simulink model "AGC"  (R2021a)
settings: Solver=FixedStepAuto  StartTime=0.0  StopTime=400  RelTol=1e-3  EnableMultiTasking=on
model workspace (MAT data in the model file):
  th = 0
libraries: dspsrcs4 x2, hdlsllib x1
settings Model: EnablePacing=on  Creator=guido  LastModifiedBy=guido
settings DataIOCC: ExternalInput=x_ts
settings OptimizationCC: BlockReduction=off  ConditionallyExecuteInputs=off  DefaultParameterBehavior=Inlined
settings DebuggingCC: SignalRangeChecking=warning  AlgebraicLoopMsg=error  SingleTaskRateTransMsg=error
settings HardwareCC: ProdBitPerPointer=32  ProdBitPerSizeT=32  ProdBitPerPtrDiffT=32  ProdLargestAtomicFloat=None  ProdIntDivRoundTo=Undefined  ProdEndianess=Unspecified  ProdWordSize=32  ProdHWDeviceType=ASIC/FPGA->ASIC/FPGA  TargetBitPerPointer=64  TargetBitPerSizeT=64  TargetBitPerPtrDiffT=64  TargetLongLongMode=on  TargetIntDivRoundTo=Zero  TargetEndianess=LittleEndian  TargetWordSize=64  TargetHWDeviceType=Custom Processor->MATLAB Host Computer  ProdEqTarget=off

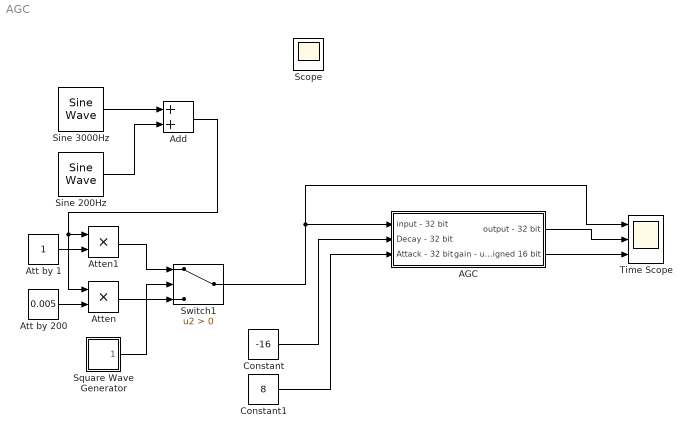
== system AGC ==
  AGC : Subsystem
  Add : Sum  AccumDataTypeStr=int32  OutDataTypeStr=int32
  Att by 1 : Constant
  Att by 200 : Constant  Value=0.005
  Atten : Product  OutDataTypeStr=int32
  Atten1 : Product  OutDataTypeStr=int32
  Constant : Constant  Value=-16  OutDataTypeStr=int32
  Constant1 : Constant  Value=8  OutDataTypeStr=int32
  Sine 200Hz : dspsrcs4/Sine Wave  Amplitude=1073741824  Frequency=200  Phase=0  SampleMode=Discrete  OutComplex=Real  CompMethod=Table lookup  TableSize=Speed  SampleTime=1/48000  SamplesPerFrame=1  ResetState=Restart at time zero  OutputFrames=off  dataType=Fixed-point  wordLen=31  udDataType=sfix(16)  fracBitsMode=Best precision  numFracBits=15  OutDataTypeStr=fixdt(1,31)  LastOutDataTypeStr=fixdt(1,31)
  Sine 3000Hz : dspsrcs4/Sine Wave  Amplitude=1073741824  Frequency=3000  Phase=0  SampleMode=Discrete  OutComplex=Real  CompMethod=Table lookup  TableSize=Speed  SampleTime=1/48000  SamplesPerFrame=1  ResetState=Restart at time zero  OutputFrames=off  dataType=Fixed-point  wordLen=31  udDataType=sfix(16)  fracBitsMode=Best precision  numFracBits=15  OutDataTypeStr=fixdt(1,31)  LastOutDataTypeStr=fixdt(1,31)
  Square Wave Generator : Subsystem  Tag=DecoupledSystem
  Switch1 : Switch  Criteria=u2 > Threshold  OutDataTypeStr=int32
  Time Scope : Scope  NumInputPorts=3
  Scope : Scope
  wires:
  Switch1/1 -> Time Scope/1, AGC/1(input - 32 bit)
  Sine 3000Hz/1 -> Add/1
  Sine 200Hz/1 -> Add/2
  Atten/1 -> Switch1/3
  Att by 200/1 -> Atten/2
  Square Wave Generator/1(Out1) -> Switch1/2
  Add/1 -> Atten1/1, Atten/1
  AGC/1(output - 32 bit) -> Time Scope/2
  AGC/2(gain - unsigned 16 bit) -> Time Scope/3
  Constant/1 -> AGC/2(Decay - 32 bit)
  Constant1/1 -> AGC/3(Attack - 32 bit)
  Atten1/1 -> Switch1/1
  Att by 1/1 -> Atten1/2

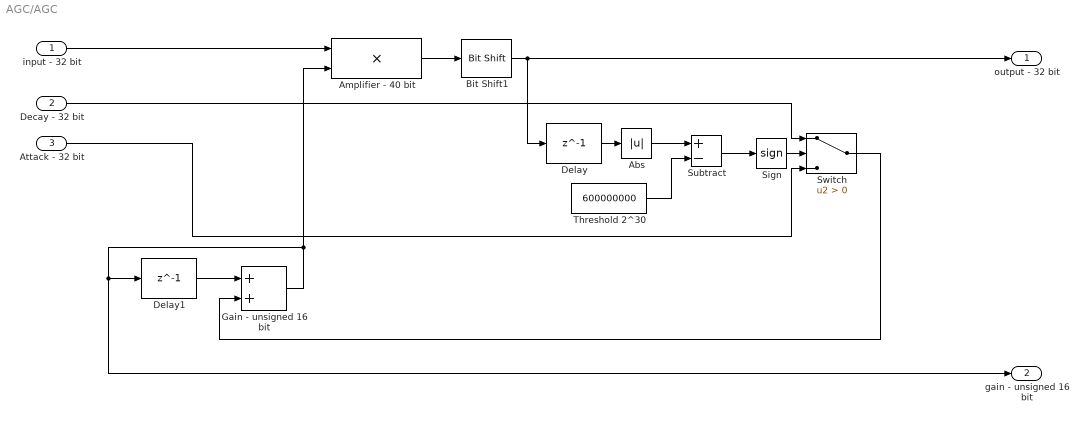
== system AGC/AGC ==
  input - 32 bit : Inport
  Decay - 32 bit : Inport  Port=2
  Attack - 32 bit : Inport  Port=3
  Abs : Abs  OutDataTypeStr=int32  SaturateOnIntegerOverflow=on
  Amplifier - 40 bit : Product  OutDataTypeStr=fixdt(1,40,0)  SaturateOnIntegerOverflow=on
  Bit Shift1 : hdlsllib/Logic and Bit Operations/Bit Shift  mode=Shift Right Arithmetic  N=8
  Delay : Delay  DelayLength=1  InitialCondition=0  UseCircularBuffer=on
  Delay1 : Delay  DelayLength=1  InitialCondition=1  UseCircularBuffer=on
  Gain - unsigned 16 bit : Sum  OutDataTypeStr=fixdt(0,16,0)  SaturateOnIntegerOverflow=on
  Sign : Signum
  Subtract : Sum  Inputs=+-  AccumDataTypeStr=int32  OutDataTypeStr=int32  SaturateOnIntegerOverflow=on
  Switch : Switch  Criteria=u2 > Threshold  OutDataTypeStr=int32  SaturateOnIntegerOverflow=on
  Threshold 2^30 : Constant  Value=600000000  OutDataTypeStr=int32
  output - 32 bit : Outport
  gain - unsigned 16 bit : Outport  Port=2
  wires:
  Delay/1 -> Abs/1
  Gain - unsigned 16 bit/1 -> Amplifier - 40 bit/2, Delay1/1, gain - unsigned 16 bit/1
  Switch/1 -> Gain - unsigned 16 bit/2
  Abs/1 -> Subtract/1
  Sign/1 -> Switch/2
  Attack - 32 bit/1 -> Switch/3
  Subtract/1 -> Sign/1
  Amplifier - 40 bit/1 -> Bit Shift1/1
  Decay - 32 bit/1 -> Switch/1
  Threshold 2^30/1 -> Subtract/2
  Delay1/1 -> Gain - unsigned 16 bit/1
  Bit Shift1/1 -> Delay/1, output - 32 bit/1
  input - 32 bit/1 -> Amplifier - 40 bit/1

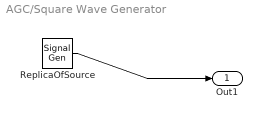
== system AGC/Square Wave Generator ==
  ReplicaOfSource : SignalGenerator  WaveForm=square  Amplitude=256  Frequency=0.5
  Out1 : Outport  LockScale=on
  wires:
  ReplicaOfSource/1 -> Out1/1
